simulink model "HapticPaddle"  (Simulink 10.1)
settings: Solver=ode4  StartTime=0.0  StopTime=30  FixedStep=0.01  RelTol=1e-3  EnableMultiTasking=on
values from neighbouring files (symbols this model uses):
  B_dash = B_p + B_m * (r_p1/r_m)^2    (= 0.000240332612223)    [Parameters.m]
  g = 9.81    [Parameters.m]
  J_dash = J_p + J_m * (r_p1/r_m)^2    (= 0.000700665224446)    [Parameters.m]
  K_dash = r_p1/r_m * k_tau    (= 0.938372093023)    [Parameters.m]
  l = 0.0199    [Parameters.m]
  m_p = 0.075    [Parameters.m]
  r_p2 = 0.065    [Parameters.m]
  s_1 = -0.4285    [Parameters.m]
  s_2 = 1.0677    [Parameters.m]
  V_0 = 2.4917    [Parameters.m]
libraries: simulink_extras x2
settings Model: Creator=jemetzge  LastModifiedBy=Administrator
settings DataIOCC: LimitDataPoints=on  SignalLoggingSaveFormat=ModelDataLogs
settings OptimizationCC: ExpressionDepthLimit=2147483647
settings DebuggingCC: SolverPrmCheckMsg=warning  FcnCallInpInsideContextMsg=warning  StateNameClashWarn=warning

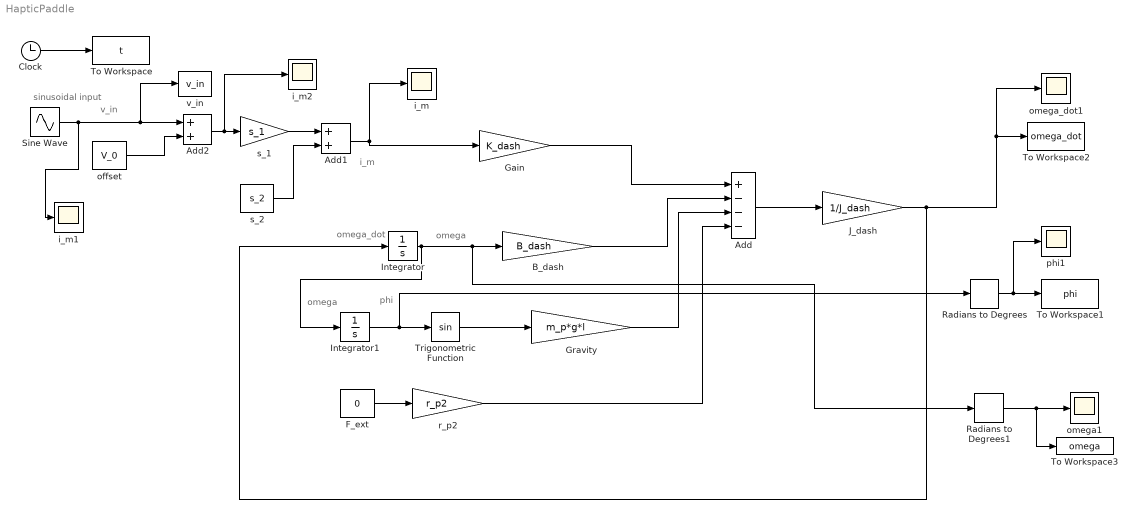
== system HapticPaddle ==
  note: omega_dot
  note: omega
  note: phi
  note: i_m
  note: v_in
  note: omega
  note: sinusoidal input
  Add : Sum  Inputs=+---
  Add1 : Sum
  Add2 : Sum
  B_dash : Gain  Gain=B_dash
  Clock : Clock
  F_ext : Constant  Value=0
  Gain : Gain  Gain=K_dash
  Gravity : Gain  Gain=m_p*g*l
  Integrator : Integrator
  Integrator1 : Integrator
  J_dash : Gain  Gain=1/J_dash
  Radians to Degrees : simulink_extras/Transformations/Radians to Degrees
  Radians to Degrees1 : simulink_extras/Transformations/Radians to Degrees
  Sine Wave : Sin  Amplitude=0.01  Frequency=2*pi*0.5  SampleTime=0
  To Workspace : ToWorkspace  VariableName=t  SampleTime=-1
  To Workspace1 : ToWorkspace  VariableName=phi  SampleTime=-1
  To Workspace2 : ToWorkspace  VariableName=omega_dot  SampleTime=-1
  To Workspace3 : ToWorkspace  VariableName=omega  SampleTime=-1
  Trigonometric Function : Trigonometry
  i_m : Scope
  i_m1 : Scope
  i_m2 : Scope
  offset : Constant  Value=V_0
  omega1 : Scope
  omega_dot1 : Scope
  phi1 : Scope
  r_p2 : Gain  Gain=r_p2
  s_1 : Gain  Gain=s_1
  s_2 : Constant  Value=s_2
  v_in : ToWorkspace  VariableName=v_in  SampleTime=-1
  wires:
  s_1/1 -> Add1/1
  s_2/1 -> Add1/2
  Add1/1 -> Gain/1, i_m/1
  F_ext/1 -> r_p2/1
  Add2/1 -> i_m2/1, s_1/1
  offset/1 -> Add2/2
  Radians to Degrees/1 -> phi1/1, To Workspace1/1
  Clock/1 -> To Workspace/1
  Radians to Degrees1/1 -> omega1/1, To Workspace3/1
  Sine Wave/1 -> i_m1/1, Add2/1, v_in/1
  Gain/1 -> Add/1
  B_dash/1 -> Add/2
  Integrator1/1 -> Radians to Degrees/1, Trigonometric Function/1
  Trigonometric Function/1 -> Gravity/1
  Gravity/1 -> Add/3
  r_p2/1 -> Add/4
  Add/1 -> J_dash/1
  Integrator/1 -> Integrator1/1, Radians to Degrees1/1, B_dash/1
  J_dash/1 -> Integrator/1, omega_dot1/1, To Workspace2/1
